simulink model "Simulink_practice"  (R2021b)
settings: Solver=ode4  StartTime=TIME.Start  StopTime=TIME.Final  FixedStep=TIME.Ts  RelTol=1e-3
values from neighbouring files (symbols this model uses):
  den = [1 2*sqrt(3)*sqrt(2) 3]    [main_simulink_practice.m]    (also in main_untitled1.m = [1 2*zt*Wn Wn^2]; main_untitled2.m = [1 0])
  Kd = 0.3    [main_simulink_practice.m]
  Ki = 1.5    [main_simulink_practice.m]
  Kp = 2.5    [main_simulink_practice.m]
  num = 3    [main_simulink_practice.m]    (also in main_untitled1.m = 144; main_untitled2.m = 1)
  TIME = struct('Ts'   , 1e-3,                'Start', 0.0 ,                'Final',20.0 ,                'stage', 0.15,                'time' , 0   ,                'Ntime', 0   )    [UAV_simulation.m]    (also in main_simulink_practice.m = struct('Start', 0.0,                'Ts'   , 1e-3,          ; main_untitled1.m = struct('Ts', 1e-3,                'Final',30,               ; main_untitled2.m = struct('Ts', 1e-3,                'Start', 0.0,             ; script_simulation.m = struct('Start', 0.0  ,                'Final',30.0  ,       )
settings Model: Creator=jinkwak  LastModifiedBy=jinkwak

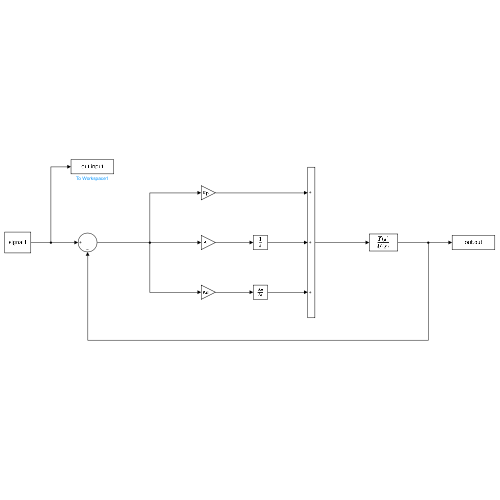
[thumbnail: Simulink's stored preview of the top-level diagram]
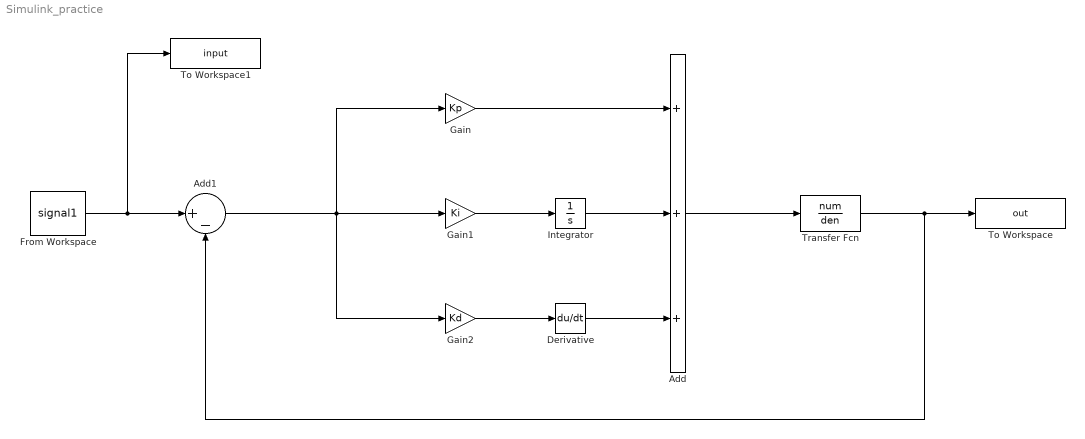
== system Simulink_practice ==
  Add : Sum  Inputs=+++
  Add1 : Sum  Inputs=|+-
  Derivative : Derivative
  From Workspace : FromWorkspace  VariableName=signal1  SampleTime=TIME.Ts
  Gain : Gain  Gain=Kp
  Gain1 : Gain  Gain=Ki
  Gain2 : Gain  Gain=Kd
  Integrator : Integrator
  To Workspace : ToWorkspace  VariableName=out  SampleTime=TIME.Ts
      settings: Save2DSignal=2-D array (concatenate along first dimension)
  To Workspace1 : ToWorkspace  VariableName=input  SampleTime=TIME.Ts
  Transfer Fcn : TransferFcn  Numerator=num  Denominator=den
  wires:
  Transfer Fcn/1 -> To Workspace/1, Add1/2
  Gain2/1 -> Derivative/1
  Add/1 -> Transfer Fcn/1
  Gain/1 -> Add/1
  Integrator/1 -> Add/2
  Gain1/1 -> Integrator/1
  Derivative/1 -> Add/3
  Add1/1 -> Gain2/1, Gain/1, Gain1/1
  From Workspace/1 -> To Workspace1/1, Add1/1
